simulink model "Subsystem10"  (R2020b)
settings: Solver=VariableStepAuto  StartTime=0.0  StopTime=10.0  RelTol=1e-3
model workspace (MAT data in the model file):
  a = Simulink.Parameter
  a.Value = 1
  a.DataType = 'auto'
  a.Dimensions = [1 1]
  b = Simulink.Parameter
  b.Value = 1
  b.DataType = 'auto'
  b.Dimensions = [1 1]
  c = Simulink.Parameter
  c.Value = 2
  c.DataType = 'auto'
  c.Dimensions = [1 1]
  d = Simulink.Parameter
  d.Value = 1
  d.DataType = 'auto'
  d.Dimensions = [1 1]
  e = Simulink.Parameter
  e.Value = -1
  e.DataType = 'auto'
  e.Dimensions = [1 1]
  f = Simulink.Parameter
  f.Value = -1
  f.DataType = 'auto'
  f.Dimensions = [1 1]
settings Model: Creator=sushma  LastModifiedBy=sushma
settings DataIOCC: SaveOutput=off  SaveTime=off

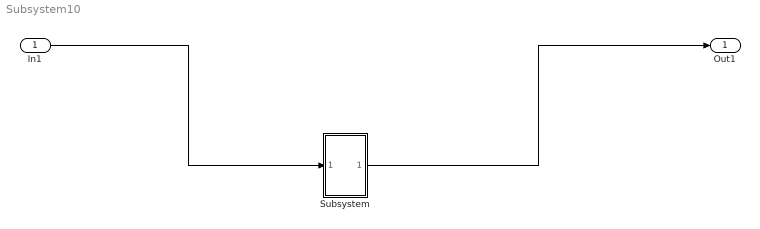
== system Subsystem10 ==
  In1 : Inport  OutDataTypeStr=double  PortDimensions=1  SampleTime=0
  Subsystem : Subsystem
  Out1 : Outport  OutDataTypeStr=double  PortDimensions=1  SampleTime=0
  wires:
  Subsystem/1(Out1) -> Out1/1
  In1/1 -> Subsystem/1(In1)

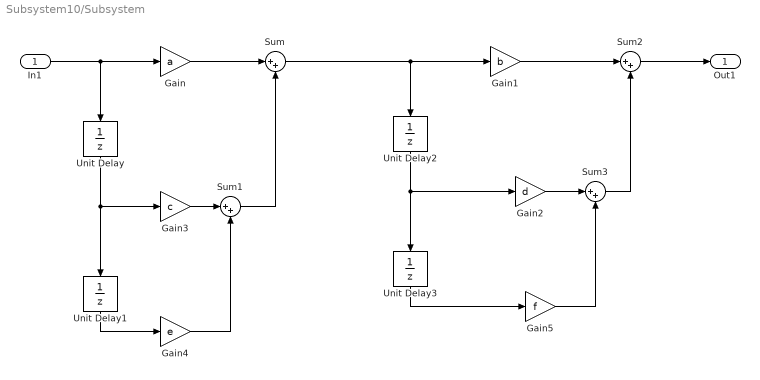
== system Subsystem10/Subsystem ==
  In1 : Inport
  Gain : Gain  Gain=a
  Gain1 : Gain  Gain=b
  Gain2 : Gain  Gain=d
  Gain3 : Gain  Gain=c
  Gain4 : Gain  Gain=e
  Gain5 : Gain  Gain=f
  Sum{,1..3} (4 alike) : Sum  Inputs=|++
  Unit Delay{,1..3} (4 alike) : UnitDelay  SampleTime=-1  HasFrameUpgradeWarning=on
  Out1 : Outport
  wires:
  Sum2/1 -> Out1/1
  Sum1/1 -> Sum/2
  Gain5/1 -> Sum3/2
  Gain4/1 -> Sum1/2
  Gain2/1 -> Sum3/1
  Unit Delay1/1 -> Gain4/1
  Gain3/1 -> Sum1/1
  Unit Delay3/1 -> Gain5/1
  Unit Delay2/1 -> Unit Delay3/1, Gain2/1
  Unit Delay/1 -> Unit Delay1/1, Gain3/1
  Gain/1 -> Sum/1
  In1/1 -> Gain/1, Unit Delay/1
  Sum/1 -> Gain1/1, Unit Delay2/1
  Gain1/1 -> Sum2/1
  Sum3/1 -> Sum2/2
